simulink model "sisreal"  (R2023b)
settings: Solver=VariableStepAuto  StartTime=0.0  StopTime=10.0  RelTol=1e-3
values from neighbouring files (symbols this model uses):
  A = 5    [Tarea_2.m]
  g = 9.81    [Tarea_2.m]
  H0 = 2.5    [Tarea_2.m]
  Kt = 3.25/100    (= 0.0325)    [Tarea_2.m]
  Kvc = Qemax/100    [Tarea_2.m]
  Kvs = 0.001    [Tarea_2.m]
  rho = 1027    [Tarea_2.m]
settings Model: Creator=roger  LastModifiedBy=roger

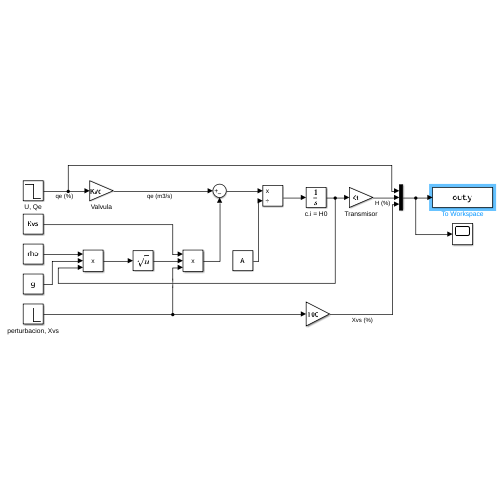
[thumbnail: Simulink's stored preview of the top-level diagram]
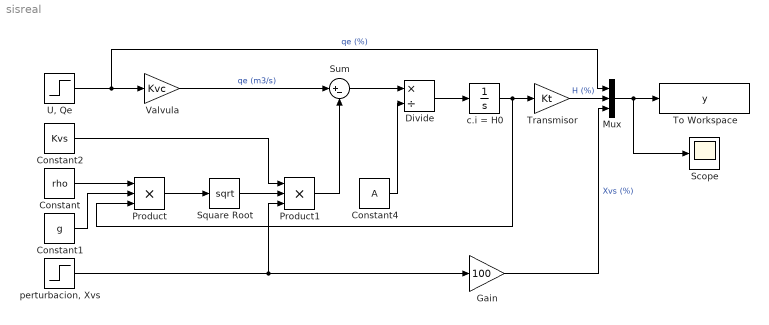
== system sisreal ==
  Constant : Constant  Value=rho
  Constant1 : Constant  Value=g
  Constant2 : Constant  Value=Kvs
  Constant4 : Constant  Value=A
  Divide : Product  Inputs=*/
  Gain : Gain  Gain=100
  Mux : Mux  Inputs=3
  Product : Product  Inputs=3
  Product1 : Product  Inputs=3
  Scope : Scope
  Square Root : Sqrt
  Sum : Sum  Inputs=|+-
  To Workspace : ToWorkspace  VariableName=y  SaveFormat=Timeseries  SampleTime=-1
  Transmisor : Gain  Gain=Kt
  "U, Qe" : Step  Before=1  After=0  SampleTime=0
  Valvula : Gain  Gain=Kvc
  c.i = H0 : Integrator  InitialCondition=H0
  "perturbacion, Xvs" : Step  Before=1  After=0  SampleTime=0
  wires:
  Constant/1 -> Product/1
  Product/1 -> Square Root/1
  Constant2/1 -> Product1/1
  Square Root/1 -> Product1/2
  "U, Qe"/1 -> Mux/1, Valvula/1  "qe (%)"
  Valvula/1 -> Sum/1  "qe (m3/s)"
  Divide/1 -> c.i = H0/1
  Product1/1 -> Sum/2
  "perturbacion, Xvs"/1 -> Product1/3, Gain/1
  c.i = H0/1 -> Product/3, Transmisor/1
  Mux/1 -> Scope/1, To Workspace/1
  Transmisor/1 -> Mux/2  "H (%)"
  Gain/1 -> Mux/3  "Xvs (%)"
  Sum/1 -> Divide/1
  Constant4/1 -> Divide/2
  Constant1/1 -> Product/2
